simulink model "PID_Kim"  (R2016a)
settings: Solver=FixedStepAuto  StartTime=0.0  StopTime=10  FixedStep=0.01  RelTol=1e-3
values from neighbouring files (symbols this model uses):
  b = 10    [Tut_Week_5.m]
  k = 20    [Tut_Week_5.m]
  M = 1    [Tut_Week_5.m]
libraries: simulink x1
settings Model: Creator=김태욱  LastModifiedBy=user
settings DataIOCC: SaveFormat=Array  SaveState=on

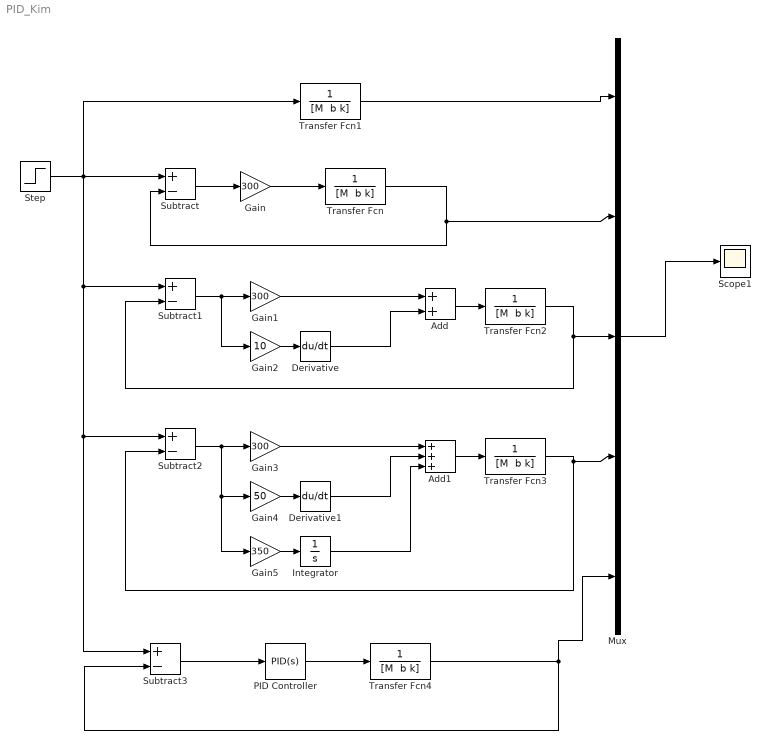
== system PID_Kim ==
  Add : Sum
  Add1 : Sum  Inputs=+++
  Derivative : Derivative
  Derivative1 : Derivative
  Gain : Gain  Gain=300
  Gain1 : Gain  Gain=300
  Gain2 : Gain  Gain=10
  Gain3 : Gain  Gain=300
  Gain4 : Gain  Gain=50
  Gain5 : Gain  Gain=350
  Integrator : Integrator
  Mux : Mux  Inputs=5
  PID Controller : simulink/Continuous/PID Controller  Controller=PID  TimeDomain=Continuous-time  SampleTime=-1  IntegratorMethod=Forward Euler  FilterMethod=Forward Euler  Form=Parallel  UseFilter=on  ControllerParametersSource=internal  P=1  I=1  D=0  N=100  InitialConditionSource=internal  InitialConditionForIntegrator=0  InitialConditionForFilter=0  ExternalReset=none  LimitOutput=off  UpperSaturationLimit=inf  LowerSaturationLimit=-inf  LinearizeAsGain=on  AntiWindupMode=none  Kb=1  TrackingMode=off  Kt=1  PParamMin=[]  PParamMax=[]  IParamMin=[]  IParamMax=[]  DParamMin=[]  DParamMax=[]  NParamMin=[]  NParamMax=[]  KbParamMin=[]  KbParamMax=[]  KtParamMin=[]  KtParamMax=[]  POutMin=[]  POutMax=[]  IOutMin=[]  IOutMax=[]  DOutMin=[]  DOutMax=[]  NOutMin=[]  NOutMax=[]  KbOutMin=[]  KbOutMax=[]  KtOutMin=[]  KtOutMax=[]  IntegratorOutMin=[]  IntegratorOutMax=[]  FilterOutMin=[]  FilterOutMax=[]  SumOutMin=[]  SumOutMax=[]  SumI1OutMin=[]  SumI1OutMax=[]  SumI2OutMin=[]  SumI2OutMax=[]  SumI3OutMin=[]  SumI3OutMax=[]  SumDOutMin=[]  SumDOutMax=[]  SaturationOutMin=[]  SaturationOutMax=[]  IntegratorContinuousStateAttributes=''  IntegratorStateMustResolveToSignalObject=off  IntegratorRTWStateStorageClass=Auto  FilterContinuousStateAttributes=''  FilterStateMustResolveToSignalObject=off  FilterRTWStateStorageClass=Auto  DifferentiatorICPrevScaledInput=0  DifferentiatorOutMin=[]  DifferentiatorOutMax=[]
  Scope1 : Scope
  Step : Step  SampleTime=0
  Subtract{,1..3} (4 alike) : Sum  Inputs=+-
  Transfer Fcn{,1..4} (5 alike) : TransferFcn  Denominator="[M  b k]"
  wires:
  Gain/1 -> Transfer Fcn/1
  Subtract/1 -> Gain/1
  Transfer Fcn/1 -> Subtract/2, Mux/2
  Transfer Fcn1/1 -> Mux/1
  Mux/1 -> Scope1/1
  Subtract1/1 -> Gain2/1, Gain1/1
  Gain2/1 -> Derivative/1
  Gain1/1 -> Add/1
  Derivative/1 -> Add/2
  Add/1 -> Transfer Fcn2/1
  Transfer Fcn2/1 -> Subtract1/2, Mux/3
  Subtract2/1 -> Gain3/1, Gain5/1, Gain4/1
  Gain4/1 -> Derivative1/1
  Gain3/1 -> Add1/1
  Derivative1/1 -> Add1/2
  Add1/1 -> Transfer Fcn3/1
  Transfer Fcn3/1 -> Subtract2/2, Mux/4
  Gain5/1 -> Integrator/1
  Integrator/1 -> Add1/3
  Step/1 -> Subtract1/1, Subtract2/1, Subtract3/1, Transfer Fcn1/1, Subtract/1
  Transfer Fcn4/1 -> Subtract3/2, Mux/5
  Subtract3/1 -> PID Controller/1
  PID Controller/1 -> Transfer Fcn4/1
